simulink model "ilc_module"  (R2024a)
settings: Solver=VariableStepAuto  StartTime=0.0  StopTime=10.0  RelTol=1e-3
settings Model: Creator=crcrisoft  LastModifiedBy=crcrisoft

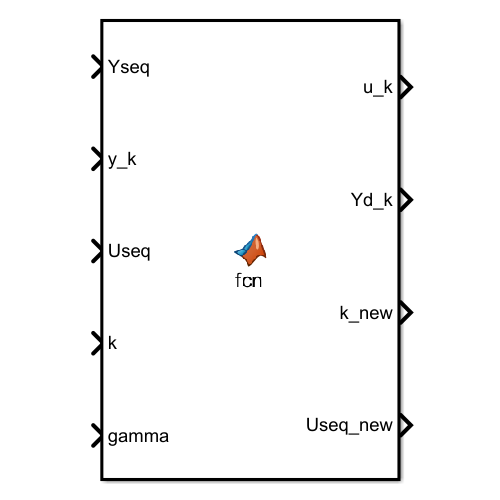
[thumbnail: Simulink's stored preview of the top-level diagram]
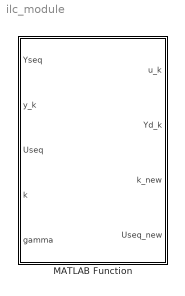
== system ilc_module ==
  MATLAB Function : MATLAB Function  TreatAsAtomicUnit=on

== matlab function ilc_module/MATLAB Function ==
  data: Yseq input; u_k output; y_k input; Useq input; k input; gamma input; Yd_k output; k_new output; Useq_new output
function [u_k,Yd_k,k_new,Useq_new] = fcn(Yseq,y_k,Useq,k,gamma)

% Yseq:
Nseq = numel(Yseq);

k_new = k+1;

if k_new > Nseq
    k_new = 1;
end

Yd_k = Yseq(k);


y = u;
